simulink model "mppt_ic"  (R2021a)
settings: Solver=VariableStepAuto  StartTime=0.0  StopTime=10.0  RelTol=1e-3
libraries: spsSeriesRLCBranchLib x3, spsDiodeLib x1, spsIGBTDiodeLib x1, spsPVArrayLib x1, eePwmGenerator x1, spsVoltageMeasurementLib x1, spspowerguiLib x1
settings Model: Creator=Dell  LastModifiedBy=Dell

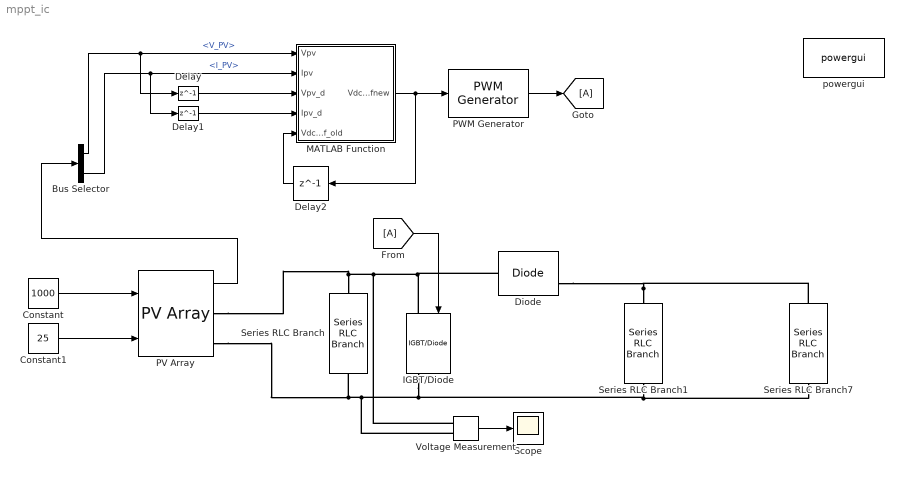
== system mppt_ic ==
  Bus Selector : BusSelector  OutputSignals=V_PV,I_PV
  Constant : Constant  Value=1000
  Constant1 : Constant  Value=25
  Delay : Delay  DelayLength=1
  Delay1 : Delay  DelayLength=1
  Delay2 : Delay  DelayLength=1  InitialCondition=1
  Diode : spsDiodeLib/Diode  Ron=0.001  Lon=0  Vf=0.8  IC=0  UseSnubber=0  Rs=500  Cs=250e-9  Measurements=on
  IGBT/Diode : spsIGBTDiodeLib/IGBT//Diode  Ron=1e-3  Rs=1e5  Cs=inf  Measurements=on
  MATLAB Function : MATLAB Function  TreatAsAtomicUnit=on
  PV Array : spsPVArrayLib/PV Array  Npar=40  Nser=10  PlotType=array @ 1000 W/m2 & specified temperatures  S_vec="[ 1000  500  100 ]"  Temp_C_vec="[ 45 25  ]"  ModuleName=User-defined  PlotWhenSelected=off  Pm=213.15  Ncell=60  Voc=36.3  Isc=7.84  Vm=29  Im=7.35  beta_Voc_pc=-0.36099  alpha_Isc_pc=0.102  beta_Voc=-0.13104  alpha_Isc=0.0079968  IL=7.8654  I0=2.9273e-10  nI=0.98119  Rsh=313.0553  Rs=0.39381  RobustModel=off  RobustCellTemperature=313.3991  BAL=on  Tc=1e-6  Tfilter=5e-5
  PWM Generator : eePwmGenerator/PWM Generator  CarrCount=Up  Tper=0.001  Ts=5e-5
  Scope : Scope
  Series RLC Branch : spsSeriesRLCBranchLib/Series RLC Branch  LConnTagsString=__new0  RConnTagsString=__new0  BranchType=C  Resistance=1  Inductance=1e-3  SetiL0=off  InitialCurrent=0  Capacitance=1e-6  Setx0=off  InitialVoltage=0  Measurements=None
  Series RLC Branch1 : spsSeriesRLCBranchLib/Series RLC Branch  LConnTagsString=__new0  RConnTagsString=__new0  BranchType=C  Resistance=1  Inductance=1e-3  SetiL0=off  InitialCurrent=0  Capacitance=1e-6  Setx0=off  InitialVoltage=0  Measurements=None
  Series RLC Branch7 : spsSeriesRLCBranchLib/Series RLC Branch  LConnTagsString=__new0  RConnTagsString=__new0  BranchType=RL  Resistance=1  Inductance=1e-3  SetiL0=off  InitialCurrent=0  Capacitance=1e-6  Setx0=off  InitialVoltage=0  Measurements=None
  Voltage Measurement : spsVoltageMeasurementLib/Voltage Measurement  PhasorSimulation=off  OutputType=Complex  PSBequivalent=0
  powergui : spspowerguiLib/powergui  Priority=1  SimulationMode=Discrete  SampleTime=50e-6  frequency=60  Iterations=50  frequencyindice=0  Pbase=100e6  ErrMax=1e-4  UnitsV=kV  UnitsW=MW  buscounter=0  FunctionMessages=off  echomessages=off  EnableUseOfTLC=off  CurrentSourceSwitches=off  DisableSnubberDevices=off  DisableRonSwitches=off  DisableVfSwitches=off  DisplayEquations=off  AutomaticDiscreteSolvers=off  SolverType=Tustin/Backward Euler (TBE)  Interpol=off  ExternalGateDelay=off  methode=off  Ts=100  x0status=blocks  SPID=on  SwTol=0  HookPort=off  NonlinearTolerance=1e-4  nMaxIteration=100  ContinueOnMaxIteration=off  RestoreLinks=warning  ResistiveCurrentMeasurement=off  Frange=[0:2:500]  Ylog=off  Xlog=on  ShowGrid=off  save=off  variable=ZData  structure=0  ZoomFFT=off  StartTime=0.0  cycles=1  DisplayStyle=1  fundamental=60  FreqAxis=off  MaxFrequency=1000  frequencyindicesteady=1  RmsSteady=1  display=off
  wires:
  Constant/1 -> PV Array/1
  Voltage Measurement/1 -> Scope/1
  PV Array/1 -> Bus Selector/1
  Constant1/1 -> PV Array/2
  MATLAB Function/1(Vdcrefnew) -> Delay2/1, PWM Generator/1
  Bus Selector/1 -> Delay/1, MATLAB Function/1(Vpv)  "<V_PV>"
  Bus Selector/2 -> Delay1/1, MATLAB Function/2(Ipv)  "<I_PV>"
  Delay/1 -> MATLAB Function/3(Vpv_d)
  Delay1/1 -> MATLAB Function/4(Ipv_d)
  PWM Generator/1 -> [A]
  [A] -> IGBT/Diode/1
  Delay2/1 -> MATLAB Function/5(Vdcref_old)
  connections:
  Series RLC Branch1/RConn1 -- PV Array/RConn2 -- Series RLC Branch/RConn1 -- Voltage Measurement/LConn2 -- IGBT/Diode/RConn1 -- Series RLC Branch7/RConn1
  Series RLC Branch1/LConn1 -- Diode/RConn1 -- Series RLC Branch7/LConn1
  IGBT/Diode/LConn1 -- Diode/LConn1 -- PV Array/RConn1 -- Series RLC Branch/LConn1 -- Voltage Measurement/LConn1

== matlab function mppt_ic/MATLAB Function ==
  data: Vpv input; Vdcrefnew output; Ipv input; Vpv_d input; Ipv_d input; Vdcref_old input
function Vdcrefnew = fcn(Vpv,Ipv,Vpv_d,Ipv_d,Vdcref_old    )
delVpv = 0.1;
delV = Vpv - Vpv_d;
delI = Ipv - Ipv_d;
if(delV == 0)
    if(delI == 0)
        Vdcrefnew = Vdcref_old;
    else
        if(delI > 0)
            Vdcrefnew = Vdcref_old + delVpv;
        else
            Vdcrefnew = Vdcref_old - delVpv;
        end
    end
else
    if((delI/delV)==(-Ipv/Vpv))
        Vdcrefnew = Vdcref_old;
    else
        if((delI/delV)>(-Ipv/Vpv))
            Vdcrefnew = Vdcref_old + delVpv;
        else
            Vdcrefnew = Vdcref_old - delVpv;
        end
    end
end
